simulink model "test_v_control_and_i_control_with_droop_copy"  (R2017b)
settings: Solver=ode3  StartTime=0.0  StopTime=10  FixedStep=1e-2  RelTol=1e-3  EnableMultiTasking=on
libraries: powerlib x43, simulink_extras x3, simulink x2
settings Model: Creator=harishsvce  LastModifiedBy=Ashwin
settings SolverCC: ConcurrentTasks=on  AutoInsertRateTranBlk=on
settings DataIOCC: MaxDataPoints=10000  SaveFormat=StructureWithTime  SignalLoggingSaveFormat=ModelDataLogs  OutputSaveName=v_out1, i_out1,v_out2, i_out2,v_out3, i_out3
settings OptimizationCC: BlockReduction=off  DefaultParameterBehavior=Inlined  OptimizeBlockIOStorage=off  BufferReuse=off  GlobalBufferReuse=off  ExpressionFolding=off  LocalBlockOutputs=off  EfficientFloat2IntCast=on
settings DebuggingCC: SaveWithParameterizedLinksMsg=none  UnderspecifiedInitializationDetection=Classic  MergeDetectMultiDrivingBlocksExec=none  SignalResolutionControl=TryResolveAllWithWarning  StateNameClashWarn=warning  SFUnexpectedBacktrackingDiag=warning  SFNoUnconditionalDefaultTransitionDiag=warning  SFExecutionAtInitializationDiag=none
settings HardwareCC: TargetBitPerPointer=64  TargetBitPerSizeT=64  TargetBitPerPtrDiffT=64  TargetLongLongMode=on  TargetIntDivRoundTo=Zero  TargetEndianess=LittleEndian  TargetWordSize=64  TargetHWDeviceType=MATLAB Host
settings ModelReferenceCC: PropagateSignalLabelsOutOfModel=off
settings RTWCC: GenCodeOnly=on  PackageGeneratedCodeAndArtifacts=on  PackageName=secondary_controller_complete_1_10_18.zip  Description=Generic Real-Time Target  GenerateReport=on  BuildConfiguration=Debug  LaunchReport=on  CodeExecutionProfiling=on  RTWCompilerOptimization=on  CheckMdlBeforeBuild=Warning
settings CodeAppCC: ForceParamTrailComments=on  MaxIdLength=95  StateflowObjectComments=on  MATLABSourceComments=on
settings GRTTargetCC: CodeReplacementLibrary=Intel IPP for x86-64 (Windows using MinGW compiler)  MultiInstanceERTCode=on  CodeInterfacePackaging=Reusable function  GenerateAllocFcn=on  RTWCAPISignals=on  RTWCAPIParams=on  RTWCAPIRootIO=on
settings ConfigComp: CovMetricSettings=dw  CovHtmlReporting=on  CovSaveCumulativeToWorkspaceVar=on  CovSaveSingleToWorkspaceVar=on  CovExternalEMLEnable=off
settings SimscapeCC: SimscapeNormalizeSystem=off  SimscapeLogType=all  SimscapeLogSimulationStatistics=on  SimscapeLogOpenViewer=on

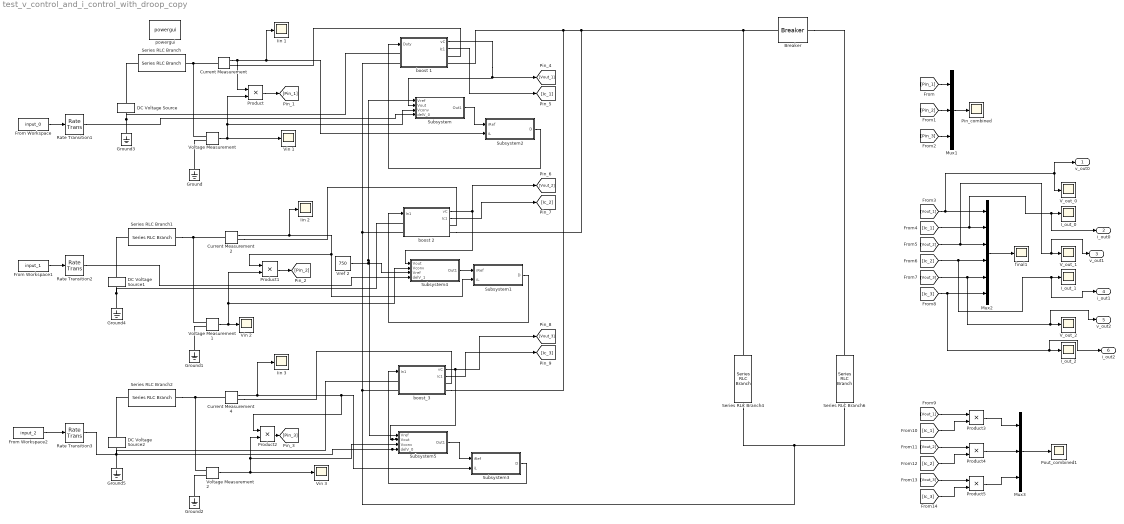
== system test_v_control_and_i_control_with_droop_copy ==
  Breaker : powerlib/Elements/Breaker  InitialState=0  SwitchingTimes=[2]  External=off  BreakerResistance=0.01  SnubberResistance=1e6  SnubberCapacitance=inf  Measurements=None  MoreParameters=on  NoBreakLoop=off
      settings: SourceProductName=Simscape Power Systems
  Current Measurement : powerlib/Measurements/Current Measurement  PhasorSimulation=off  OutputType=Complex  PSBequivalent=0
  Current Measurement2 : powerlib/Measurements/Current Measurement  PhasorSimulation=off  OutputType=Complex  PSBequivalent=0
  Current Measurement4 : powerlib/Measurements/Current Measurement  PhasorSimulation=off  OutputType=Complex  PSBequivalent=0
  DC Voltage Source : powerlib/Electrical Sources/DC Voltage Source  Amplitude=200  Measurements=None
  DC Voltage Source1 : powerlib/Electrical Sources/DC Voltage Source  Amplitude=200  Measurements=None
  DC Voltage Source2 : powerlib/Electrical Sources/DC Voltage Source  Amplitude=200  Measurements=None
  From Workspace : FromWorkspace  VariableName=input_0  SampleTime=0.01
  From Workspace1 : FromWorkspace  VariableName=input_1  SampleTime=0.01
  From Workspace2 : FromWorkspace  VariableName=input_2  SampleTime=0.01
  Ground{,1..5} (6 alike) : powerlib/Elements/Ground  LConnTagsString=a
  I_out_0 : Scope
  I_out_1 : Scope
  I_out_2 : Scope
  Iin 1 : Scope
  Iin 2 : Scope
  Iin 3 : Scope
  Mux1 : Mux  Inputs=3
  Mux2 : Mux  Inputs=6
  Mux3 : Mux  Inputs=3
  Pin_combined : Scope
  Pout_combined1 : Scope
  Product{,1..5} (6 alike) : Product
  Rate Transition1 : RateTransition  OutPortSampleTime=0.01
  Rate Transition2 : RateTransition  OutPortSampleTime=0.01
  Rate Transition3 : RateTransition  OutPortSampleTime=0.01
  Series RLC Branch : powerlib/Elements/Series RLC Branch  LConnTagsString=__new0  RConnTagsString=__new0  BranchType=R  Resistance=0.001  Inductance=0  SetiL0=on  InitialCurrent=0  Capacitance=1e-6  Setx0=off  InitialVoltage=0  Measurements=None
  Series RLC Branch1 : powerlib/Elements/Series RLC Branch  LConnTagsString=__new0  RConnTagsString=__new0  BranchType=R  Resistance=0.001  Inductance=0  SetiL0=on  InitialCurrent=0  Capacitance=1e-6  Setx0=off  InitialVoltage=0  Measurements=None
  Series RLC Branch2 : powerlib/Elements/Series RLC Branch  LConnTagsString=__new0  RConnTagsString=__new0  BranchType=R  Resistance=0.001  Inductance=0  SetiL0=on  InitialCurrent=0  Capacitance=1e-6  Setx0=off  InitialVoltage=0  Measurements=None
  Series RLC Branch4 : powerlib/Elements/Series RLC Branch  LConnTagsString=__new0  RConnTagsString=__new0  BranchType=R  Resistance=28.125*2  Inductance=5e-3  SetiL0=on  InitialCurrent=0  Capacitance=1e-6  Setx0=off  InitialVoltage=0  Measurements=None
  Series RLC Branch6 : powerlib/Elements/Series RLC Branch  LConnTagsString=__new0  RConnTagsString=__new0  BranchType=R  Resistance=56.25*2  Inductance=5e-3  SetiL0=on  InitialCurrent=0  Capacitance=1e-6  Setx0=off  InitialVoltage=0  Measurements=None
  Subsystem : Subsystem
  Subsystem1 : Subsystem
  Subsystem2 : Subsystem
  Subsystem3 : Subsystem
  Subsystem4 : Subsystem
  Subsystem5 : Subsystem
  V_out_0 : Scope
  V_out_1 : Scope
  V_out_2 : Scope
  Vin 1 : Scope
  Vin 2 : Scope
  Vin 3 : Scope
  Voltage Measurement : powerlib/Measurements/Voltage Measurement  PhasorSimulation=off  OutputType=Complex  PSBequivalent=0
  Voltage Measurement1 : powerlib/Measurements/Voltage Measurement  PhasorSimulation=off  OutputType=Complex  PSBequivalent=0
  Voltage Measurement2 : powerlib/Measurements/Voltage Measurement  PhasorSimulation=off  OutputType=Complex  PSBequivalent=0
  Vref 2 : Constant  Value=750
  "boost 1 " : Subsystem
  boost 2 : Subsystem
  boost_3 : Subsystem
  final1 : Scope
  powergui : powerlib/powergui  Priority=1  SimulationMode=Discrete  SampleTime=1e-2  frequency=60  Iterations=50  frequencyindice=0  Pbase=100e6  ErrMax=1e-4  UnitsV=kV  UnitsW=MW  buscounter=0  FunctionMessages=off  echomessages=off  EnableUseOfTLC=off  CurrentSourceSwitches=off  DisableSnubberDevices=off  DisableRonSwitches=off  DisableVfSwitches=off  DisplayEquations=off  SolverType=Tustin/Backward Euler (TBE)  Interpol=off  ExternalGateDelay=off  methode=off  Ts=10  x0status=blocks  SPID=on  SwTol=0  HookPort=off  RestoreLinks=warning  ResistiveCurrentMeasurement=off  Frange=[0:2:500]  Ylog=off  Xlog=on  ShowGrid=off  save=off  variable=ZData  structure=0  ZoomFFT=off  StartTime=0.0  cycles=1  DisplayStyle=1  fundamental=60  FreqAxis=off  MaxFrequency=1000  frequencyindicesteady=1  RmsSteady=1  display=off
  v_out0 : Outport
  i_out0 : Outport  Port=2
  v_out1 : Outport  Port=3
  i_out1 : Outport  Port=4
  v_out2 : Outport  Port=5
  i_out2 : Outport  Port=6
  wires:
  Current Measurement/1 -> Subsystem2/2(iL), Iin 1/1, Product/1
  "boost 1 "/1(vC) -> Subsystem/2(Vout), [Vout_1]
  Current Measurement4/1 -> Subsystem3/2(iL), Product2/1, Iin 3/1
  Vref 2/1 -> Subsystem5/1(Vref), Subsystem/1(Vref), Subsystem4/3(Vref)
  "boost 1 "/2(Ic1) -> [Ic_1]
  boost 2/2(Ic1) -> [Ic_2]
  boost_3/2(Ic1) -> [Ic_3]
  boost 2/1(vC) -> Subsystem4/1(Vout), [Vout_2]
  Subsystem/1(Out1) -> Subsystem2/1("iRef ")
  Subsystem2/1("D ") -> "boost 1 "/1(Duty)
  Subsystem4/1(Out1) -> Subsystem1/1("iRef ")
  Subsystem1/1("D ") -> boost 2/1(In1)
  Subsystem5/1(Out1) -> Subsystem3/1("iRef ")
  Subsystem3/1("D ") -> boost_3/1(In1)
  Voltage Measurement2/1 -> Subsystem5/3(Vconv), Product2/2, Vin 3/1
  Current Measurement2/1 -> Subsystem1/2(iL), Product1/1, Iin 2/1
  Voltage Measurement1/1 -> Subsystem4/2(Vconv), Product1/2, Vin 2/1
  Product/1 -> [Pin_1]
  [Pin_1] -> Mux1/1
  [Pin_2] -> Mux1/2
  [Pin_3] -> Mux1/3
  Product1/1 -> [Pin_2]
  Product2/1 -> [Pin_3]
  Voltage Measurement/1 -> Vin 1/1, Subsystem/3(Vconv), Product/2
  Mux1/1 -> Pin_combined/1
  [Vout_1] -> V_out_0/1, v_out0/1, Mux2/1
  [Ic_1] -> i_out0/1, I_out_0/1, Mux2/2
  [Vout_2] -> v_out1/1, V_out_1/1, Mux2/3
  [Ic_2] -> i_out1/1, I_out_1/1, Mux2/4
  [Vout_3] -> v_out2/1, V_out_2/1, Mux2/5
  [Ic_3] -> i_out2/1, I_out_2/1, Mux2/6
  Mux2/1 -> final1/1
  [Vout_1] -> Product3/1
  [Ic_1] -> Product3/2
  [Vout_2] -> Product4/1
  [Ic_2] -> Product4/2
  [Vout_3] -> Product5/1
  [Ic_3] -> Product5/2
  Product4/1 -> Mux3/2
  Product3/1 -> Mux3/1
  Product5/1 -> Mux3/3
  Mux3/1 -> Pout_combined1/1
  From Workspace/1 -> Rate Transition1/1
  Rate Transition1/1 -> Subsystem/4(delV_0)
  From Workspace2/1 -> Rate Transition3/1
  From Workspace1/1 -> Rate Transition2/1
  Rate Transition2/1 -> Subsystem4/4(delV_1)
  Rate Transition3/1 -> Subsystem5/4(delV_0)
  boost_3/1(vC) -> Subsystem5/2(Vout), [Vout_3]
  connections:
  Series RLC Branch/LConn1 -- Voltage Measurement/LConn1 -- Current Measurement/LConn1
  DC Voltage Source/LConn1 -- "boost 1 "/LConn1 -- Ground3/LConn1
  DC Voltage Source1/LConn1 -- boost 2/LConn1 -- Ground4/LConn1
  DC Voltage Source2/LConn1 -- boost_3/LConn1 -- Ground5/LConn1
  boost 2/RConn2 -- Series RLC Branch4/RConn1 -- Breaker/LConn1 -- boost_3/RConn2 -- "boost 1 "/RConn2
  boost 2/LConn2 -- boost_3/LConn2 -- Series RLC Branch6/LConn1 -- Series RLC Branch4/LConn1 -- "boost 1 "/LConn2
  Series RLC Branch1/LConn1 -- Voltage Measurement1/LConn1 -- Current Measurement2/LConn1
  Ground2/LConn1 -- Voltage Measurement2/LConn2
  Series RLC Branch2/LConn1 -- Voltage Measurement2/LConn1 -- Current Measurement4/LConn1
  Ground/LConn1 -- Voltage Measurement/LConn2
  DC Voltage Source/RConn1 -- Series RLC Branch/RConn1
  Current Measurement/RConn1 -- "boost 1 "/RConn1
  Ground1/LConn1 -- Voltage Measurement1/LConn2
  Current Measurement2/RConn1 -- boost 2/RConn1
  DC Voltage Source2/RConn1 -- Series RLC Branch2/RConn1
  DC Voltage Source1/RConn1 -- Series RLC Branch1/RConn1
  Current Measurement4/RConn1 -- boost_3/RConn1
  Breaker/RConn1 -- Series RLC Branch6/RConn1

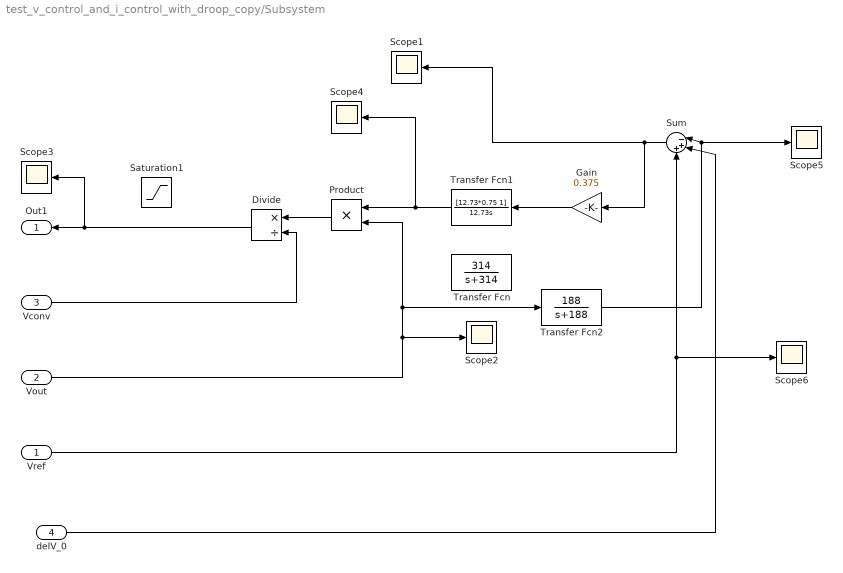
== system test_v_control_and_i_control_with_droop_copy/Subsystem ==
  Vref : Inport
  Vout : Inport  Port=2
  Vconv : Inport  Port=3
  delV_0 : Inport  Port=4
  Divide : Product  Inputs=*/
  Gain : Gain  Gain=0.375
  Product : Product
  Saturation1 : Saturate  UpperLimit=45  LowerLimit=-0.1
  Scope{1..6} (6 alike) : Scope
  Sum : Sum  Inputs=|-++
  Transfer Fcn : TransferFcn  Numerator=[314]  Denominator=[1 314]
  Transfer Fcn1 : TransferFcn  Numerator=[12.73*0.75 1]  Denominator=[12.73 0]
  Transfer Fcn2 : TransferFcn  Numerator=[188]  Denominator=[1 188]
  Out1 : Outport
  wires:
  Sum/1 -> Scope1/1, Gain/1
  Vref/1 -> Sum/3, Scope6/1
  Product/1 -> Divide/1
  Transfer Fcn1/1 -> Scope4/1, Product/1
  Gain/1 -> Transfer Fcn1/1
  Divide/1 -> Scope3/1, Out1/1
  Vconv/1 -> Divide/2
  Vout/1 -> Transfer Fcn2/1, Product/2, Scope2/1
  Transfer Fcn2/1 -> Scope5/1, Sum/1
  delV_0/1 -> Sum/2

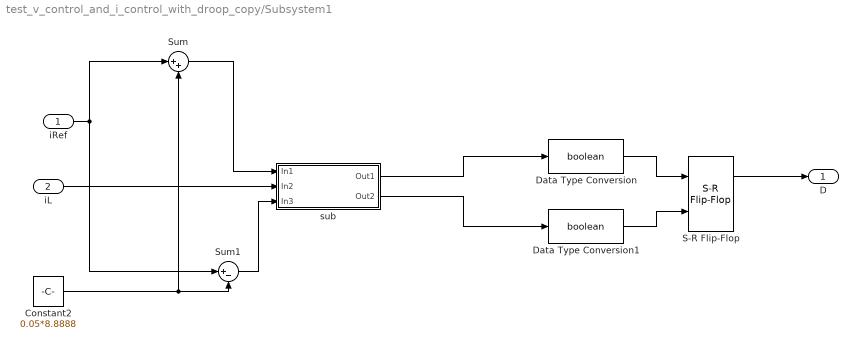
== system test_v_control_and_i_control_with_droop_copy/Subsystem1 ==
  "iRef " : Inport
  iL : Inport  Port=2
  Constant2 : Constant  Value=0.05*8.8888
  Data Type Conversion : DataTypeConversion  OutDataTypeStr=boolean  SaturateOnIntegerOverflow=on
  Data Type Conversion1 : DataTypeConversion  OutDataTypeStr=boolean
  S-R Flip-Flop : simulink_extras/Flip Flops/S-R Flip-Flop  initial_condition=0
  Sum : Sum  Inputs=|++
  Sum1 : Sum  Inputs=|+-
  "sub " : Subsystem
  "D " : Outport
  wires:
  Data Type Conversion/1 -> S-R Flip-Flop/1
  Data Type Conversion1/1 -> S-R Flip-Flop/2
  S-R Flip-Flop/1 -> "D "/1
  "sub "/1(Out1) -> Data Type Conversion/1
  "sub "/2(Out2) -> Data Type Conversion1/1
  Constant2/1 -> Sum1/2, Sum/2
  Sum/1 -> "sub "/1(In1)
  Sum1/1 -> "sub "/3(In3)
  "iRef "/1 -> Sum1/1, Sum/1
  iL/1 -> "sub "/2(In2)

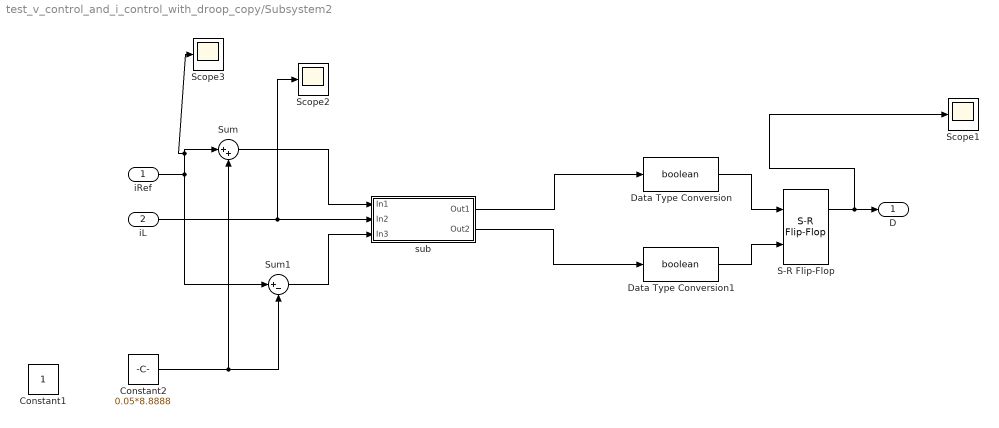
== system test_v_control_and_i_control_with_droop_copy/Subsystem2 ==
  "iRef " : Inport
  iL : Inport  Port=2
  Constant1 : Constant
  Constant2 : Constant  Value=0.05*8.8888
  Data Type Conversion : DataTypeConversion  OutDataTypeStr=boolean  SaturateOnIntegerOverflow=on
  Data Type Conversion1 : DataTypeConversion  OutDataTypeStr=boolean
  S-R Flip-Flop : simulink_extras/Flip Flops/S-R Flip-Flop  initial_condition=0
  Scope1 : Scope
  Scope2 : Scope
  Scope3 : Scope
  Sum : Sum  Inputs=|++
  Sum1 : Sum  Inputs=|+-
  "sub " : Subsystem
  "D " : Outport
  wires:
  Data Type Conversion/1 -> S-R Flip-Flop/1
  Data Type Conversion1/1 -> S-R Flip-Flop/2
  S-R Flip-Flop/1 -> Scope1/1, "D "/1
  "sub "/1(Out1) -> Data Type Conversion/1
  "sub "/2(Out2) -> Data Type Conversion1/1
  Constant2/1 -> Sum1/2, Sum/2
  Sum/1 -> "sub "/1(In1)
  Sum1/1 -> "sub "/3(In3)
  "iRef "/1 -> Sum1/1, Scope3/1, Sum/1
  iL/1 -> Scope2/1, "sub "/2(In2)

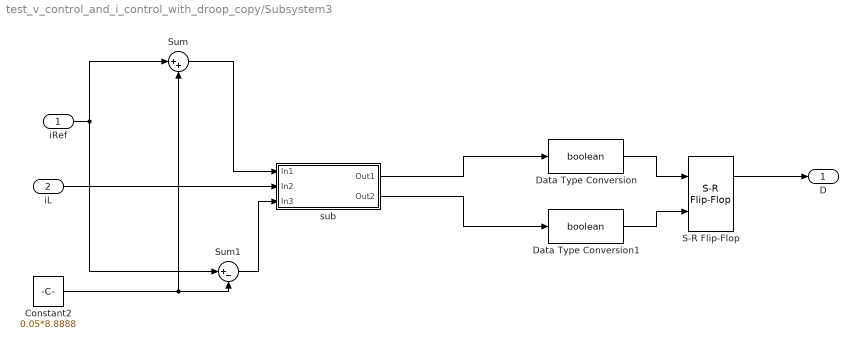
== system test_v_control_and_i_control_with_droop_copy/Subsystem3 ==
  "iRef " : Inport
  iL : Inport  Port=2
  Constant2 : Constant  Value=0.05*8.8888
  Data Type Conversion : DataTypeConversion  OutDataTypeStr=boolean  SaturateOnIntegerOverflow=on
  Data Type Conversion1 : DataTypeConversion  OutDataTypeStr=boolean
  S-R Flip-Flop : simulink_extras/Flip Flops/S-R Flip-Flop  initial_condition=0
  Sum : Sum  Inputs=|++
  Sum1 : Sum  Inputs=|+-
  "sub " : Subsystem
  "D " : Outport
  wires:
  Data Type Conversion/1 -> S-R Flip-Flop/1
  Data Type Conversion1/1 -> S-R Flip-Flop/2
  S-R Flip-Flop/1 -> "D "/1
  "sub "/1(Out1) -> Data Type Conversion/1
  "sub "/2(Out2) -> Data Type Conversion1/1
  Constant2/1 -> Sum1/2, Sum/2
  Sum/1 -> "sub "/1(In1)
  Sum1/1 -> "sub "/3(In3)
  "iRef "/1 -> Sum1/1, Sum/1
  iL/1 -> "sub "/2(In2)

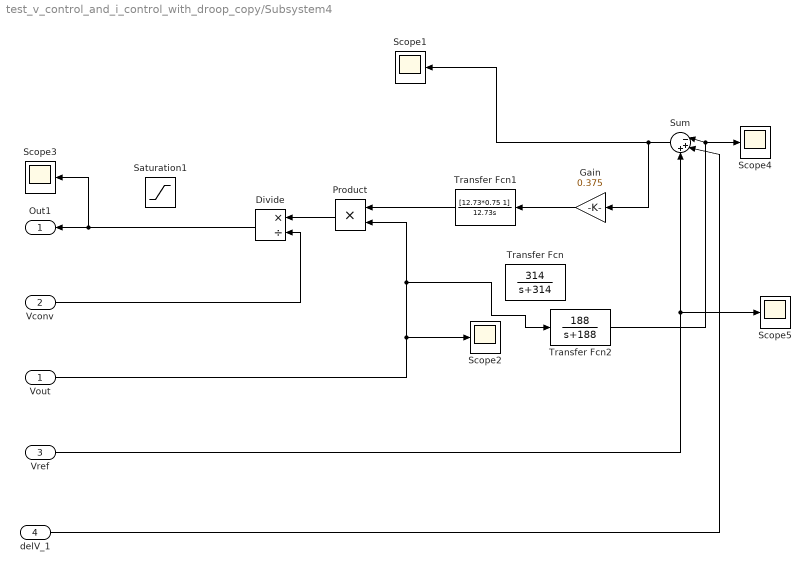
== system test_v_control_and_i_control_with_droop_copy/Subsystem4 ==
  Vout : Inport
  Vconv : Inport  Port=2
  Vref : Inport  Port=3
  delV_1 : Inport  Port=4
  Divide : Product  Inputs=*/
  Gain : Gain  Gain=0.375
  Product : Product
  Saturation1 : Saturate  UpperLimit=45  LowerLimit=-0.1
  Scope{1..5} (5 alike) : Scope
  Sum : Sum  Inputs=|-++
  Transfer Fcn : TransferFcn  Numerator=[314]  Denominator=[1 314]
  Transfer Fcn1 : TransferFcn  Numerator=[12.73*0.75 1]  Denominator=[12.73 0]
  Transfer Fcn2 : TransferFcn  Numerator=[188]  Denominator=[1 188]
  Out1 : Outport
  wires:
  Sum/1 -> Scope1/1, Gain/1
  Vref/1 -> Sum/3, Scope5/1
  Product/1 -> Divide/1
  Transfer Fcn1/1 -> Product/1
  Gain/1 -> Transfer Fcn1/1
  Divide/1 -> Scope3/1, Out1/1
  Vout/1 -> Transfer Fcn2/1, Product/2, Scope2/1
  Vconv/1 -> Divide/2
  Transfer Fcn2/1 -> Scope4/1, Sum/1
  delV_1/1 -> Sum/2

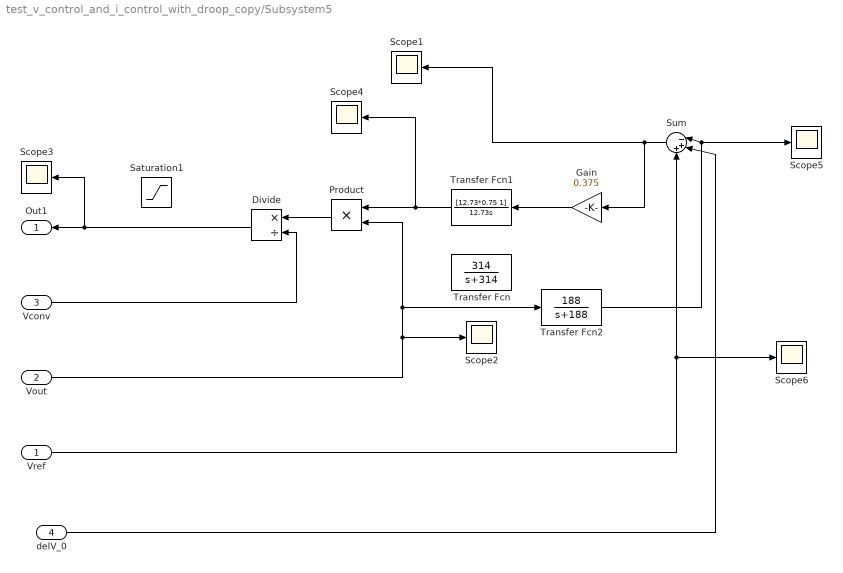
== system test_v_control_and_i_control_with_droop_copy/Subsystem5 ==
  Vref : Inport
  Vout : Inport  Port=2
  Vconv : Inport  Port=3
  delV_0 : Inport  Port=4
  Divide : Product  Inputs=*/
  Gain : Gain  Gain=0.375
  Product : Product
  Saturation1 : Saturate  UpperLimit=45  LowerLimit=-0.1
  Scope{1..6} (6 alike) : Scope
  Sum : Sum  Inputs=|-++
  Transfer Fcn : TransferFcn  Numerator=[314]  Denominator=[1 314]
  Transfer Fcn1 : TransferFcn  Numerator=[12.73*0.75 1]  Denominator=[12.73 0]
  Transfer Fcn2 : TransferFcn  Numerator=[188]  Denominator=[1 188]
  Out1 : Outport
  wires:
  delV_0/1 -> Sum/2
  Transfer Fcn2/1 -> Scope5/1, Sum/1
  Vconv/1 -> Divide/2
  Divide/1 -> Scope3/1, Out1/1
  Sum/1 -> Scope1/1, Gain/1
  Product/1 -> Divide/1
  Vout/1 -> Transfer Fcn2/1, Product/2, Scope2/1
  Vref/1 -> Sum/3, Scope6/1
  Gain/1 -> Transfer Fcn1/1
  Transfer Fcn1/1 -> Scope4/1, Product/1

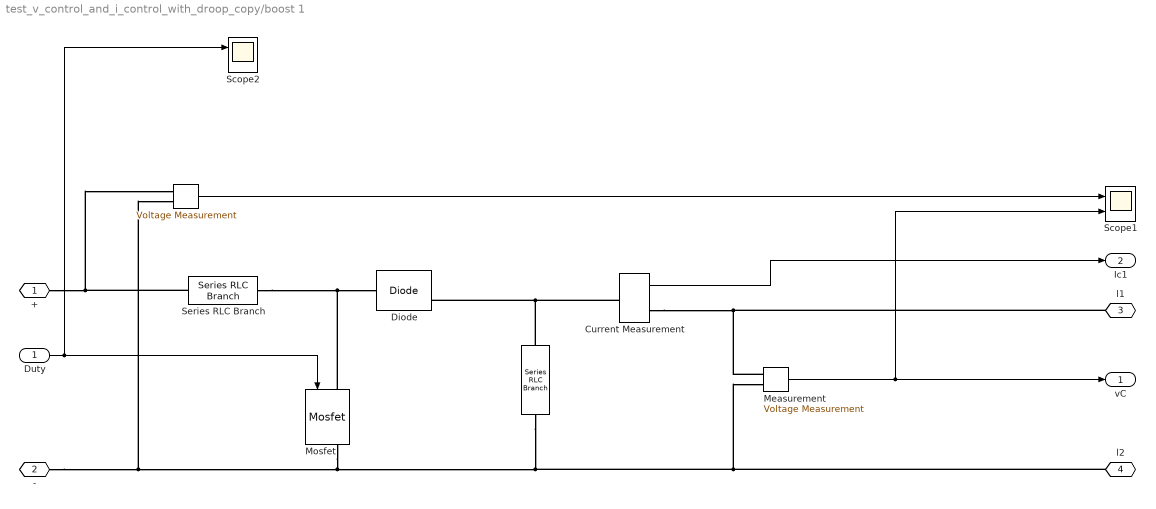
== system test_v_control_and_i_control_with_droop_copy/boost 1  ==
  Duty : Inport
  "  " : powerlib/Measurements/Voltage Measurement  PhasorSimulation=off  OutputType=Complex  PSBequivalent=0
  "    " : powerlib/Elements/Series RLC Branch  LConnTagsString=__new0  RConnTagsString=__new0  BranchType=C  Resistance=0  Inductance=69e-3  SetiL0=off  InitialCurrent=0  Capacitance=17e-3  Setx0=off  InitialVoltage=0  Measurements=None
  " Measurement" : powerlib/Measurements/Voltage Measurement  PhasorSimulation=off  OutputType=Complex  PSBequivalent=0
  Current Measurement : powerlib/Measurements/Current Measurement  PhasorSimulation=off  OutputType=Complex  PSBequivalent=0
  Diode : powerlib/Power Electronics/Diode  Ron=0.001  Lon=0  Vf=0.8  IC=0  UseSnubber=off  Rs=500  Cs=250e-9  Measurements=on
  Mosfet : powerlib/Power Electronics/Mosfet  Ron=0.1  Lon=0  Rd=0.01  Vfd=0  IC=0  Rs=1e5  Cs=inf  Measurements=on
  Scope1 : Scope  NumInputPorts=2
  Scope2 : Scope  NumInputPorts=2
  Series RLC Branch : powerlib/Elements/Series RLC Branch  LConnTagsString=__new0  RConnTagsString=__new0  BranchType=L  Resistance=0  Inductance=80e-3  SetiL0=off  InitialCurrent=0  Capacitance=1e-6  Setx0=off  InitialVoltage=0  Measurements=None
  + : PMIOPort  Port=1  Side=Right
  "- " : PMIOPort  Port=2  Side=Left
  l1 : PMIOPort  Port=3  Side=Right
  l2 : PMIOPort  Port=4  Side=Left
  vC : Outport
  Ic1 : Outport  Port=2
  wires:
  Current Measurement/1 -> Ic1/1
  " Measurement"/1 -> vC/1, Scope1/2
  "  "/1 -> Scope1/1
  Duty/1 -> Scope2/1, Mosfet/1
  connections:
  "    "/RConn1 -- l2/RConn1 -- " Measurement"/LConn2 -- Mosfet/RConn1 -- "- "/RConn1 -- "  "/LConn2
  Current Measurement/LConn1 -- "    "/LConn1 -- Diode/RConn1
  Series RLC Branch/LConn1 -- +/RConn1 -- "  "/LConn1
  Mosfet/LConn1 -- Diode/LConn1 -- Series RLC Branch/RConn1
  " Measurement"/LConn1 -- l1/RConn1 -- Current Measurement/RConn1

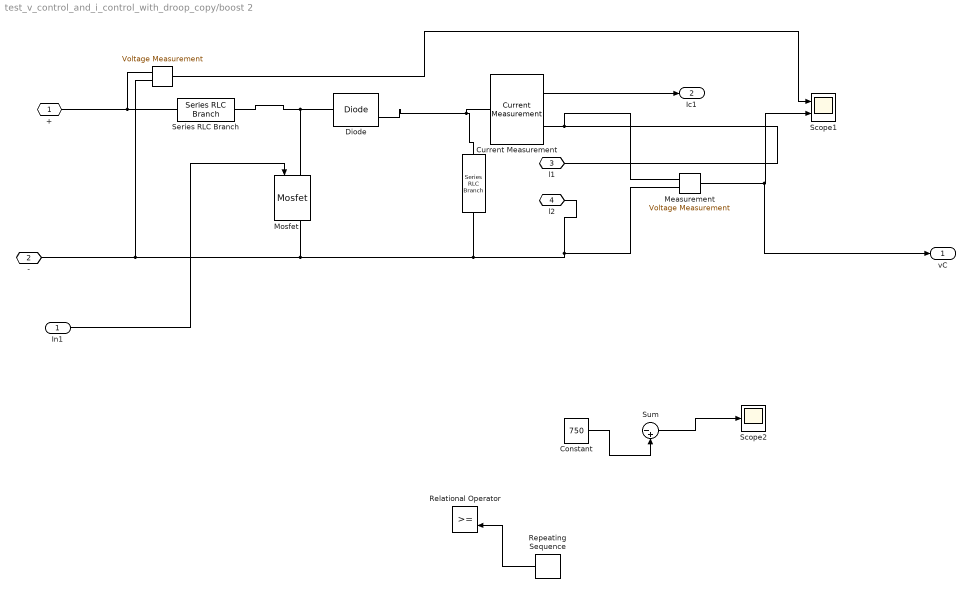
== system test_v_control_and_i_control_with_droop_copy/boost 2 ==
  In1 : Inport
  "  " : powerlib/Measurements/Voltage Measurement  PhasorSimulation=off  OutputType=Complex  PSBequivalent=0
  "    " : powerlib/Elements/Series RLC Branch  LConnTagsString=__new0  RConnTagsString=__new0  BranchType=C  Resistance=0  Inductance=69e-3  SetiL0=off  InitialCurrent=0  Capacitance=17e-3  Setx0=off  InitialVoltage=0  Measurements=None
  " Measurement" : powerlib/Measurements/Voltage Measurement  PhasorSimulation=off  OutputType=Complex  PSBequivalent=0
  Constant : Constant  Value=750
  Current Measurement : powerlib/Measurements/Current Measurement  PhasorSimulation=off  OutputType=Complex  PSBequivalent=0
  Diode : powerlib/Power Electronics/Diode  Ron=0.001  Lon=0  Vf=0.8  IC=0  UseSnubber=off  Rs=500  Cs=250e-9  Measurements=on
  Mosfet : powerlib/Power Electronics/Mosfet  Ron=0.1  Lon=0  Rd=0.01  Vfd=0  IC=0  Rs=1e5  Cs=inf  Measurements=on
  Relational Operator : RelationalOperator  OutDataTypeStr=boolean  RndMeth=Nearest
  Repeating Sequence : simulink/Sources/Repeating Sequence  rep_seq_t=[0 0.00005 0.0001]  rep_seq_y=[0 1 0]
  Scope1 : Scope  NumInputPorts=2
  Scope2 : Scope
  Series RLC Branch : powerlib/Elements/Series RLC Branch  LConnTagsString=__new0  RConnTagsString=__new0  BranchType=L  Resistance=0  Inductance=80e-3  SetiL0=off  InitialCurrent=0  Capacitance=1e-6  Setx0=off  InitialVoltage=0  Measurements=None
  Sum : Sum  Inputs=|-+
  + : PMIOPort  Port=1  Side=Right
  "- " : PMIOPort  Port=2  Side=Left
  "l1 " : PMIOPort  Port=3  Side=Right
  "l2 " : PMIOPort  Port=4  Side=Left
  vC : Outport
  Ic1 : Outport  Port=2
  wires:
  Current Measurement/1 -> Ic1/1
  " Measurement"/1 -> vC/1, Scope1/2
  "  "/1 -> Scope1/1
  Constant/1 -> Sum/2
  Sum/1 -> Scope2/1
  Repeating Sequence/1 -> Relational Operator/2
  In1/1 -> Mosfet/1
  connections:
  " Measurement"/LConn2 -- "    "/RConn1 -- Mosfet/RConn1 -- "- "/RConn1 -- "  "/LConn2 -- "l2 "/RConn1
  Diode/RConn1 -- "    "/LConn1 -- Current Measurement/LConn1
  Series RLC Branch/LConn1 -- "  "/LConn1 -- +/RConn1
  Mosfet/LConn1 -- Diode/LConn1 -- Series RLC Branch/RConn1
  " Measurement"/LConn1 -- Current Measurement/RConn1 -- "l1 "/RConn1

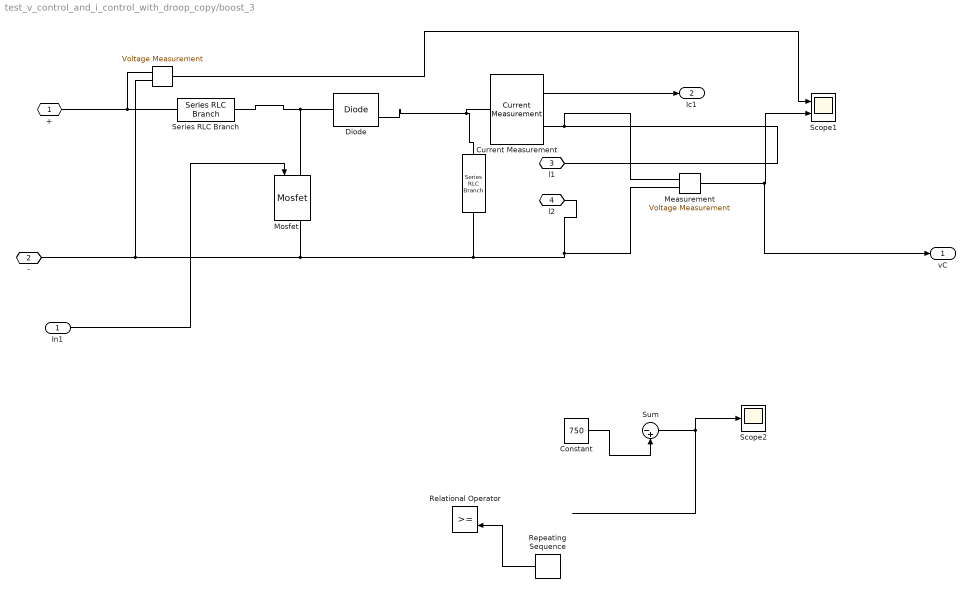
== system test_v_control_and_i_control_with_droop_copy/boost_3 ==
  In1 : Inport
  "  " : powerlib/Measurements/Voltage Measurement  PhasorSimulation=off  OutputType=Complex  PSBequivalent=0
  "    " : powerlib/Elements/Series RLC Branch  LConnTagsString=__new0  RConnTagsString=__new0  BranchType=C  Resistance=0  Inductance=69e-3  SetiL0=off  InitialCurrent=0  Capacitance=17e-3  Setx0=off  InitialVoltage=0  Measurements=None
  " Measurement" : powerlib/Measurements/Voltage Measurement  PhasorSimulation=off  OutputType=Complex  PSBequivalent=0
  Constant : Constant  Value=750
  Current Measurement : powerlib/Measurements/Current Measurement  PhasorSimulation=off  OutputType=Complex  PSBequivalent=0
  Diode : powerlib/Power Electronics/Diode  Ron=0.001  Lon=0  Vf=0.8  IC=0  UseSnubber=off  Rs=500  Cs=250e-9  Measurements=on
  Mosfet : powerlib/Power Electronics/Mosfet  Ron=0.1  Lon=0  Rd=0.01  Vfd=0  IC=0  Rs=1e5  Cs=inf  Measurements=on
  Relational Operator : RelationalOperator  OutDataTypeStr=boolean  RndMeth=Nearest
  Repeating Sequence : simulink/Sources/Repeating Sequence  rep_seq_t=[0 0.00005 0.0001]  rep_seq_y=[0 1 0]
  Scope1 : Scope  NumInputPorts=2
  Scope2 : Scope
  Series RLC Branch : powerlib/Elements/Series RLC Branch  LConnTagsString=__new0  RConnTagsString=__new0  BranchType=L  Resistance=0  Inductance=80e-3  SetiL0=off  InitialCurrent=0  Capacitance=1e-6  Setx0=off  InitialVoltage=0  Measurements=None
  Sum : Sum  Inputs=|-+
  + : PMIOPort  Port=1  Side=Right
  "- " : PMIOPort  Port=2  Side=Left
  "l1 " : PMIOPort  Port=3  Side=Right
  "l2 " : PMIOPort  Port=4  Side=Left
  vC : Outport
  Ic1 : Outport  Port=2
  wires:
  Current Measurement/1 -> Ic1/1
  " Measurement"/1 -> vC/1, Scope1/2
  "  "/1 -> Scope1/1
  Constant/1 -> Sum/2
  Sum/1 -> Scope2/1
  Repeating Sequence/1 -> Relational Operator/2
  ? -> Relational Operator/1
  In1/1 -> Mosfet/1
  connections:
  " Measurement"/LConn2 -- "    "/RConn1 -- Mosfet/RConn1 -- "- "/RConn1 -- "  "/LConn2 -- "l2 "/RConn1
  Diode/RConn1 -- "    "/LConn1 -- Current Measurement/LConn1
  Series RLC Branch/LConn1 -- "  "/LConn1 -- +/RConn1
  Mosfet/LConn1 -- Diode/LConn1 -- Series RLC Branch/RConn1
  " Measurement"/LConn1 -- Current Measurement/RConn1 -- "l1 "/RConn1

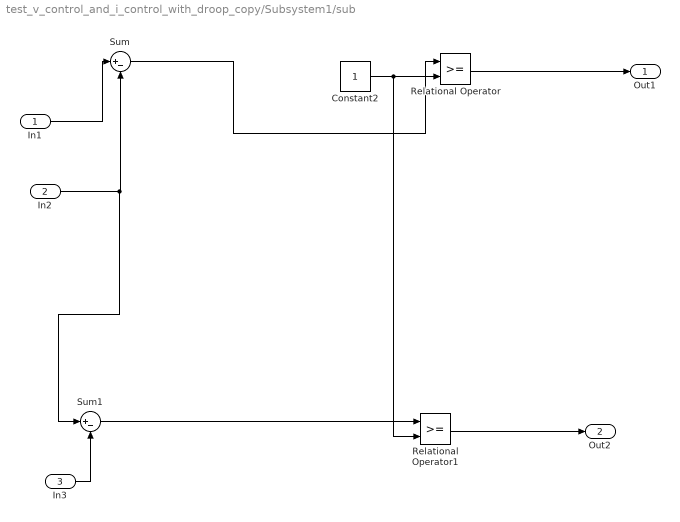
== system test_v_control_and_i_control_with_droop_copy/Subsystem1/sub  ==
  In1 : Inport
  In2 : Inport  Port=2
  In3 : Inport  Port=3
  Constant2 : Constant
  Relational Operator : RelationalOperator  OutDataTypeStr=boolean  RndMeth=Nearest
  Relational Operator1 : RelationalOperator  OutDataTypeStr=boolean  RndMeth=Nearest
  Sum : Sum  Inputs=|+-
  Sum1 : Sum  Inputs=|+-
  Out1 : Outport
  Out2 : Outport  Port=2
  wires:
  In2/1 -> Sum1/1, Sum/2
  In1/1 -> Sum/1
  Relational Operator/1 -> Out1/1
  Relational Operator1/1 -> Out2/1
  Sum/1 -> Relational Operator/1
  Sum1/1 -> Relational Operator1/1
  Constant2/1 -> Relational Operator1/2, Relational Operator/2
  In3/1 -> Sum1/2

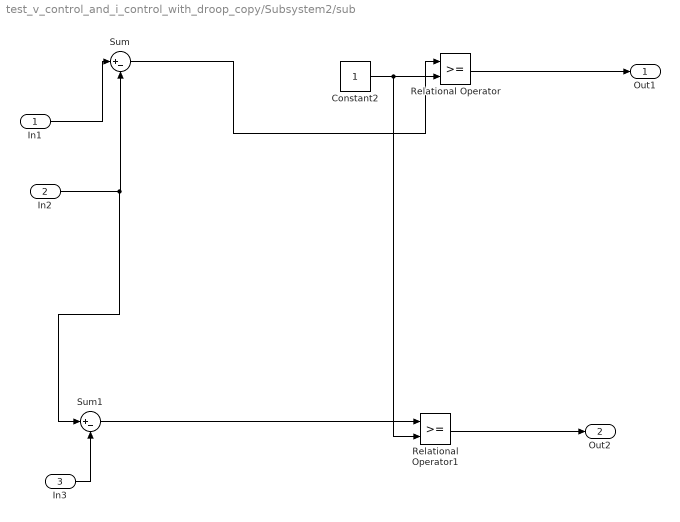
== system test_v_control_and_i_control_with_droop_copy/Subsystem2/sub  ==
  In1 : Inport
  In2 : Inport  Port=2
  In3 : Inport  Port=3
  Constant2 : Constant
  Relational Operator : RelationalOperator  OutDataTypeStr=boolean  RndMeth=Nearest
  Relational Operator1 : RelationalOperator  OutDataTypeStr=boolean  RndMeth=Nearest
  Sum : Sum  Inputs=|+-
  Sum1 : Sum  Inputs=|+-
  Out1 : Outport
  Out2 : Outport  Port=2
  wires:
  In2/1 -> Sum1/1, Sum/2
  In1/1 -> Sum/1
  Relational Operator/1 -> Out1/1
  Relational Operator1/1 -> Out2/1
  Sum/1 -> Relational Operator/1
  Sum1/1 -> Relational Operator1/1
  Constant2/1 -> Relational Operator1/2, Relational Operator/2
  In3/1 -> Sum1/2

== system test_v_control_and_i_control_with_droop_copy/Subsystem3/sub  ==
  In1 : Inport
  In2 : Inport  Port=2
  In3 : Inport  Port=3
  Constant2 : Constant
  Relational Operator : RelationalOperator  OutDataTypeStr=boolean  RndMeth=Nearest
  Relational Operator1 : RelationalOperator  OutDataTypeStr=boolean  RndMeth=Nearest
  Sum : Sum  Inputs=|+-
  Sum1 : Sum  Inputs=|+-
  Out1 : Outport
  Out2 : Outport  Port=2
  wires:
  In2/1 -> Sum1/1, Sum/2
  In1/1 -> Sum/1
  Relational Operator/1 -> Out1/1
  Relational Operator1/1 -> Out2/1
  Sum/1 -> Relational Operator/1
  Sum1/1 -> Relational Operator1/1
  Constant2/1 -> Relational Operator1/2, Relational Operator/2
  In3/1 -> Sum1/2
